simulink model "satellite_model"  (R2024a)
settings: Solver=ode4  StartTime=0.0  StopTime=1500  FixedStep=0.001  RelTol=1e-7  AbsTol=1e-7
values from neighbouring files (symbols this model uses):
  a1 = 5e-6    (= 5e-06)    [quadcopter_param.m]    (also in satellite_param.m = ab1 / I(1,1); unicycle_param.m = 4e-05)
  a2 = 7.5e-6    (= 7.5e-06)    [quadcopter_param.m]    (also in satellite_param.m = ab2 / I(2,2); unicycle_param.m = 0.0052)
  a3 = 8.5e-6    (= 8.5e-06)    [quadcopter_param.m]    (also in satellite_param.m = ab3 / I(3,3))
  a4 = ab1 / -IRW(1,1)    [satellite_param.m]
  a5 = ab2 / -IRW(2,2)    [satellite_param.m]
  a6 = ab3 / -IRW(3,3)    [satellite_param.m]
  c1 = 0.154    [quadcopter_param.m]    (also in satellite_param.m = cb1 / I(1,1); unicycle_param.m = 0.4)
  c2 = 0.237    [quadcopter_param.m]    (also in satellite_param.m = cb2 / I(2,2); unicycle_param.m = 2.4)
  c3 = 0.185    [quadcopter_param.m]    (also in satellite_param.m = cb3 / I(3,3))
  c4 = cb1 / -IRW(1,1)    [satellite_param.m]
  c5 = cb2 / -IRW(2,2)    [satellite_param.m]
  c6 = cb3 / -IRW(3,3)    [satellite_param.m]
  delay = 0.01    [quadcopter_param.m]    (also in satellite_param.m = 0.003; unicycle_param.m)
  k = 3.95    [quadcopter_param.m]    (also in satellite_param.m = 2.4; unicycle_param.m = 12.5)
  omega = 25    [quadcopter_param.m]    (also in satellite_param.m = 36; unicycle_param.m = 50)
  variance = 1e-6    (= 1e-06)    [quadcopter_param.m]    (also in satellite_param.m = 1e-09; unicycle_param.m)
settings Model: Creator=rohan  LastModifiedBy=rohan

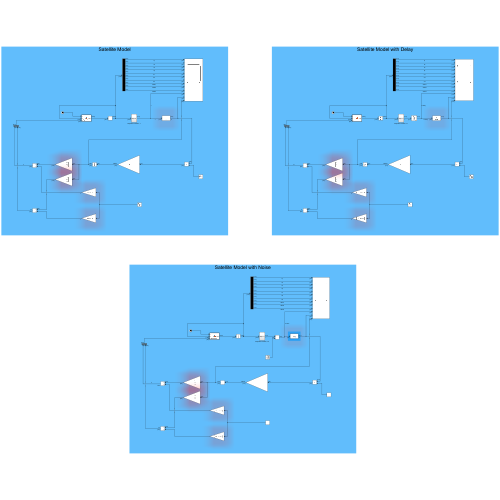
[thumbnail: Simulink's stored preview of the top-level diagram]
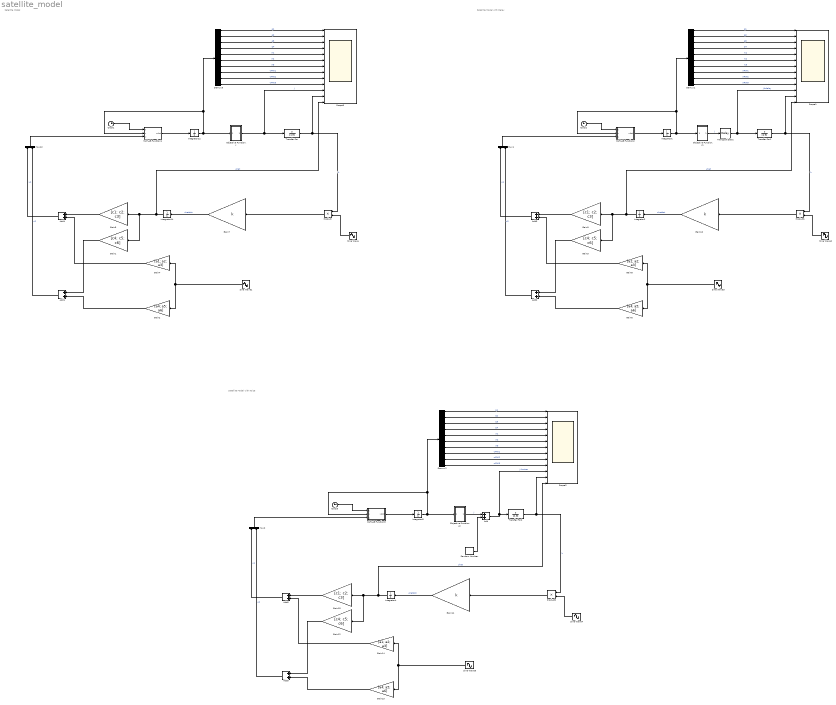
== system satellite_model ==
  note: Satellite Model
  note: Satellite Model with Delay
  note: Satellite Model with Noise
  Add{,1..6} (7 alike) : Sum
  Clock1 : Clock
  Clock2 : Clock
  Clock3 : Clock
  Demux1 : Demux  Outputs=10
  Demux2 : Demux  Outputs=10
  Demux5 : Demux  Outputs=10
  Gain1 : Gain  Gain=[c4; c5; c6]
  Gain10 : Gain  Gain=k
  Gain11 : Gain  Gain=k
  Gain12 : Gain  Gain=[c4; c5; c6]
  Gain13 : Gain  Gain=[a4; a5; a6]
  Gain14 : Gain  Gain=[a1; a2; a3]
  Gain15 : Gain  Gain=[c1; c2; c3]
  Gain2 : Gain  Gain=[a4; a5; a6]
  Gain3 : Gain  Gain=[c4; c5; c6]
  Gain4 : Gain  Gain=[a1; a2; a3]
  Gain5 : Gain  Gain=[c1; c2; c3]
  Gain6 : Gain  Gain=[a4; a5; a6]
  Gain7 : Gain  Gain=k
  Gain8 : Gain  Gain=[a1; a2; a3]
  Gain9 : Gain  Gain=[c1; c2; c3]
  Integrator1 : Integrator  InitialCondition=[0.57; 0.57; 0.57; 0.159; 0.01; 0.01; 0.01; 0; 0; 0]
  Integrator12 : Integrator  InitialCondition=[0.57; 0.57; 0.57; 0.159; 0.01; 0.01; 0.01; 0; 0; 0]
  Integrator14 : Integrator
  Integrator2 : Integrator
  Integrator3 : Integrator  InitialCondition=[0.57; 0.57; 0.57; 0.159; 0.01; 0.01; 0.01; 0; 0; 0]
  Integrator4 : Integrator
  MATLAB Function1 : MATLAB Function  TreatAsAtomicUnit=on
  MATLAB Function2 : MATLAB Function  TreatAsAtomicUnit=on
  MATLAB Function3 : MATLAB Function  TreatAsAtomicUnit=on
  Mux1 : Mux  Inputs=2
  Mux12 : Mux  Inputs=2
  Mux2 : Mux  Inputs=2
  "Objective Function, J" : Subsystem
  "Objective Function, J1" : Subsystem
  "Objective Function, J2" : Subsystem
  Product : Product
  Product1 : Product
  Product2 : Product
  Random Number : RandomNumber  Variance=variance  Seed=1  SampleTime=0.001
  Scope1 : Scope  NumInputPorts=13
  Scope2 : Scope  NumInputPorts=13
  Scope3 : Scope  NumInputPorts=13
  Sine Wave{,1..5} (6 alike) : Sin  Amplitude=omega  Frequency=omega  Phase=pi/2  SampleTime=0
  Transfer Fcn : TransferFcn  Numerator=[1 0]  Denominator=[1 e]
  Transfer Fcn1 : TransferFcn  Numerator=[1 0]  Denominator=[1 e]
  Transfer Fcn2 : TransferFcn  Numerator=[1 0]  Denominator=[1 e]
  Transport Delay : TransportDelay  DelayTime=delay  InitialOutput=3 * (0.57 - 0)^2
  wires:
  MATLAB Function1/1(xdot) -> Integrator12/1
  Integrator12/1 -> MATLAB Function1/2(x), Demux5/1, "Objective Function, J"/1(In2)
  Clock1/1 -> MATLAB Function1/1(t)
  "Objective Function, J"/1(objFun1) -> Transfer Fcn/1, Scope3/11  "J"
  Add4/1 -> Mux12/1  "u1"
  Gain4/1 -> Add4/2
  Integrator14/1 -> Scope3/13, Gain1/1, Gain5/1  "uhat"
  Gain5/1 -> Add4/1
  Sine Wave1/1 -> Gain4/1, Gain2/1
  Sine Wave/1 -> Product/2
  Gain7/1 -> Integrator14/1  "uhatdot"
  Gain1/1 -> Add1/1
  Gain2/1 -> Add1/2
  Add1/1 -> Mux12/2  "u2"
  Mux12/1 -> MATLAB Function1/3(u)
  Demux5/1 -> Scope3/1  "q1"
  Demux5/2 -> Scope3/2  "q2"
  Demux5/3 -> Scope3/3  "q3"
  Demux5/4 -> Scope3/4  "q4"
  Demux5/5 -> Scope3/5  "w1"
  Demux5/6 -> Scope3/6  "w2"
  Demux5/7 -> Scope3/7  "w3"
  Demux5/8 -> Scope3/8  "wRW1"
  Demux5/9 -> Scope3/9  "wRW2"
  Demux5/10 -> Scope3/10  "wRW3"
  Product/1 -> Gain7/1
  Transfer Fcn/1 -> Product/1, Scope3/12  "h"
  Sine Wave2/1 -> Product1/2
  Mux1/1 -> MATLAB Function2/3(u)
  Add2/1 -> Mux1/2  "u2"
  Gain9/1 -> Add3/1
  Gain6/1 -> Add2/2
  Demux1/4 -> Scope1/4  "q4"
  Demux1/9 -> Scope1/9  "wRW2"
  Integrator2/1 -> Scope1/13, Gain3/1, Gain9/1  "uhat"
  Demux1/1 -> Scope1/1  "q1"
  Transfer Fcn1/1 -> Product1/1, Scope1/12  "h"
  Product1/1 -> Gain10/1
  Demux1/7 -> Scope1/7  "w3"
  Demux1/8 -> Scope1/8  "wRW1"
  Demux1/3 -> Scope1/3  "q3"
  Gain3/1 -> Add2/1
  Gain8/1 -> Add3/2
  Demux1/5 -> Scope1/5  "w1"
  Add3/1 -> Mux1/1  "u1"
  "Objective Function, J1"/1(objFun1) -> Transport Delay/1  "J"
  Gain10/1 -> Integrator2/1  "uhatdot"
  Demux1/2 -> Scope1/2  "q2"
  Demux1/10 -> Scope1/10  "wRW3"
  Clock2/1 -> MATLAB Function2/1(t)
  Demux1/6 -> Scope1/6  "w2"
  Integrator1/1 -> MATLAB Function2/2(x), Demux1/1, "Objective Function, J1"/1(In2)
  MATLAB Function2/1(xdot) -> Integrator1/1
  Sine Wave3/1 -> Gain8/1, Gain6/1
  Sine Wave5/1 -> Gain13/1, Gain14/1
  MATLAB Function3/1(xdot) -> Integrator3/1
  Integrator3/1 -> "Objective Function, J2"/1(In2), Demux2/1, MATLAB Function3/2(x)
  Demux2/6 -> Scope2/6  "w2"
  Clock3/1 -> MATLAB Function3/1(t)
  Demux2/10 -> Scope2/10  "wRW3"
  Demux2/2 -> Scope2/2  "q2"
  Gain11/1 -> Integrator4/1  "uhatdot"
  Add6/1 -> Mux2/1  "u1"
  Demux2/5 -> Scope2/5  "w1"
  Gain14/1 -> Add6/2
  Gain12/1 -> Add5/1
  Demux2/3 -> Scope2/3  "q3"
  Demux2/8 -> Scope2/8  "wRW1"
  Demux2/7 -> Scope2/7  "w3"
  Product2/1 -> Gain11/1
  Transfer Fcn2/1 -> Scope2/12, Product2/1  "h"
  Demux2/1 -> Scope2/1  "q1"
  Integrator4/1 -> Scope2/13, Gain15/1, Gain12/1  "uhat"
  Demux2/9 -> Scope2/9  "wRW2"
  Demux2/4 -> Scope2/4  "q4"
  Gain13/1 -> Add5/2
  Gain15/1 -> Add6/1
  Add5/1 -> Mux2/2  "u2"
  Mux2/1 -> MATLAB Function3/3(u)
  Sine Wave4/1 -> Product2/2
  Transport Delay/1 -> Transfer Fcn1/1, Scope1/11  "J+delay"
  "Objective Function, J2"/1(objFun1) -> Add/1  "J"
  Add/1 -> Transfer Fcn2/1, Scope2/11  "J+noise"
  Random Number/1 -> Add/2

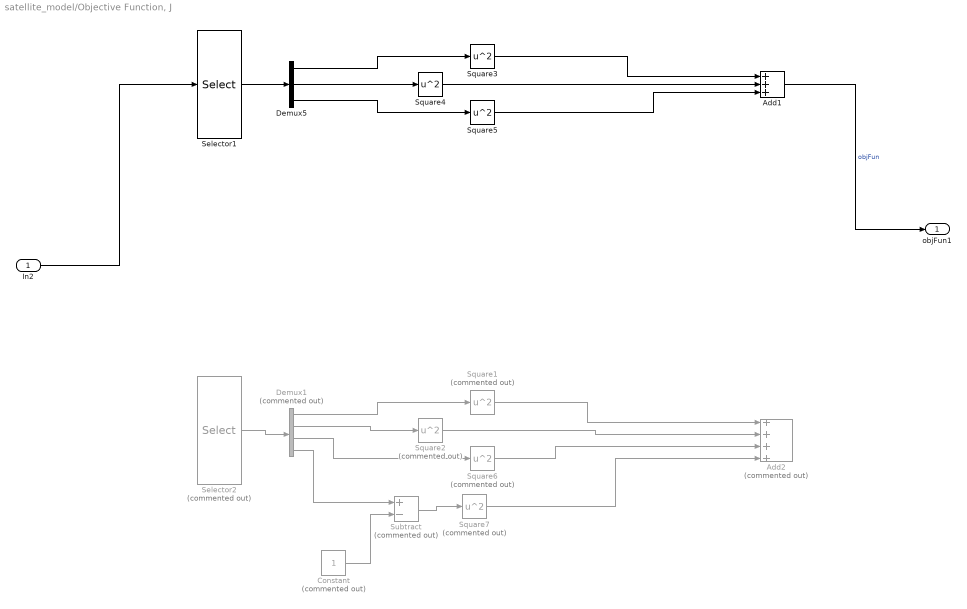
== system satellite_model/Objective Function, J ==
  In2 : Inport
  Add1 : Sum  Inputs=+++
  Add2 : Sum  Commented=on  Inputs=++++
  Constant : Constant  Commented=on
  Demux1 : Demux  Commented=on
  Demux5 : Demux  Outputs=3
  Selector1 : Selector  InputPortWidth=10  IndexOptions=Index vector (dialog)  Indices=[1 2 3]  OutputSizes=1
  Selector2 : Selector  Commented=on  InputPortWidth=10  IndexOptions=Index vector (dialog)  Indices=[1 2 3 4]  OutputSizes=1
  Square{1..2,6..7} (4 alike) : Math  Commented=on  Operator=square
  Square3 : Math  Operator=square
  Square4 : Math  Operator=square
  Square5 : Math  Operator=square
  Subtract : Sum  Commented=on  Inputs=+-
  objFun1 : Outport
  wires:
  Square4/1 -> Add1/2
  Demux5/2 -> Square4/1
  Square5/1 -> Add1/3
  Demux5/1 -> Square3/1
  Selector1/1 -> Demux5/1
  Square3/1 -> Add1/1
  Demux5/3 -> Square5/1
  Demux1/3 -> Square6/1
  Square1/1 -> Add2/1
  Selector2/1 -> Demux1/1
  Demux1/1 -> Square1/1
  Square6/1 -> Add2/3
  Demux1/2 -> Square2/1
  Square2/1 -> Add2/2
  Demux1/4 -> Subtract/1
  Constant/1 -> Subtract/2
  Subtract/1 -> Square7/1
  Square7/1 -> Add2/4
  In2/1 -> Selector1/1
  Add1/1 -> objFun1/1  "objFun"

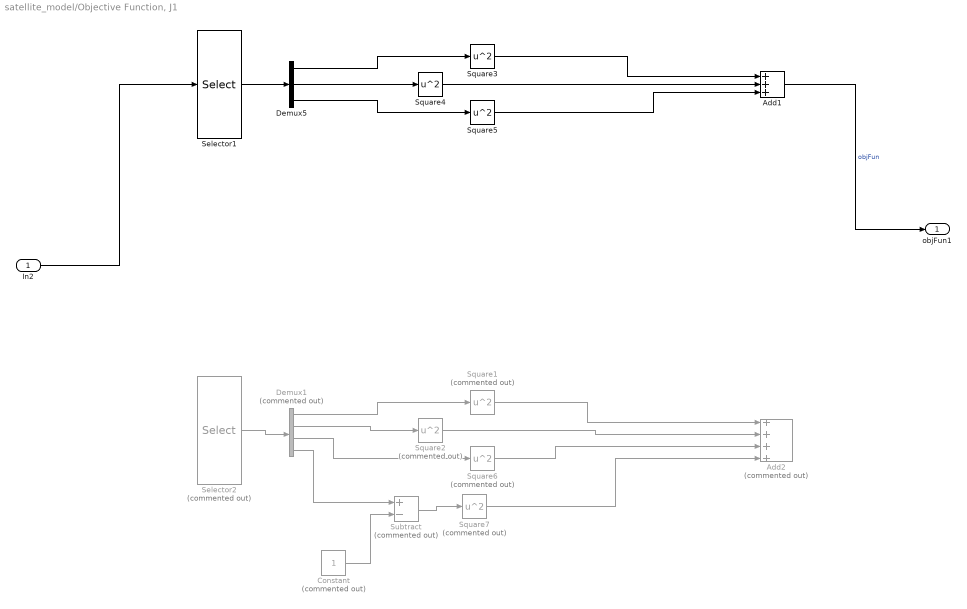
== system satellite_model/Objective Function, J1 ==
  In2 : Inport
  Add1 : Sum  Inputs=+++
  Add2 : Sum  Commented=on  Inputs=++++
  Constant : Constant  Commented=on
  Demux1 : Demux  Commented=on
  Demux5 : Demux  Outputs=3
  Selector1 : Selector  InputPortWidth=10  IndexOptions=Index vector (dialog)  Indices=[1 2 3]  OutputSizes=1
  Selector2 : Selector  Commented=on  InputPortWidth=10  IndexOptions=Index vector (dialog)  Indices=[1 2 3 4]  OutputSizes=1
  Square{1..2,6..7} (4 alike) : Math  Commented=on  Operator=square
  Square3 : Math  Operator=square
  Square4 : Math  Operator=square
  Square5 : Math  Operator=square
  Subtract : Sum  Commented=on  Inputs=+-
  objFun1 : Outport
  wires:
  Square4/1 -> Add1/2
  Demux5/2 -> Square4/1
  Square5/1 -> Add1/3
  Demux5/1 -> Square3/1
  Selector1/1 -> Demux5/1
  Square3/1 -> Add1/1
  Demux5/3 -> Square5/1
  Demux1/3 -> Square6/1
  Square1/1 -> Add2/1
  Selector2/1 -> Demux1/1
  Demux1/1 -> Square1/1
  Square6/1 -> Add2/3
  Demux1/2 -> Square2/1
  Square2/1 -> Add2/2
  Demux1/4 -> Subtract/1
  Constant/1 -> Subtract/2
  Subtract/1 -> Square7/1
  Square7/1 -> Add2/4
  In2/1 -> Selector1/1
  Add1/1 -> objFun1/1  "objFun"

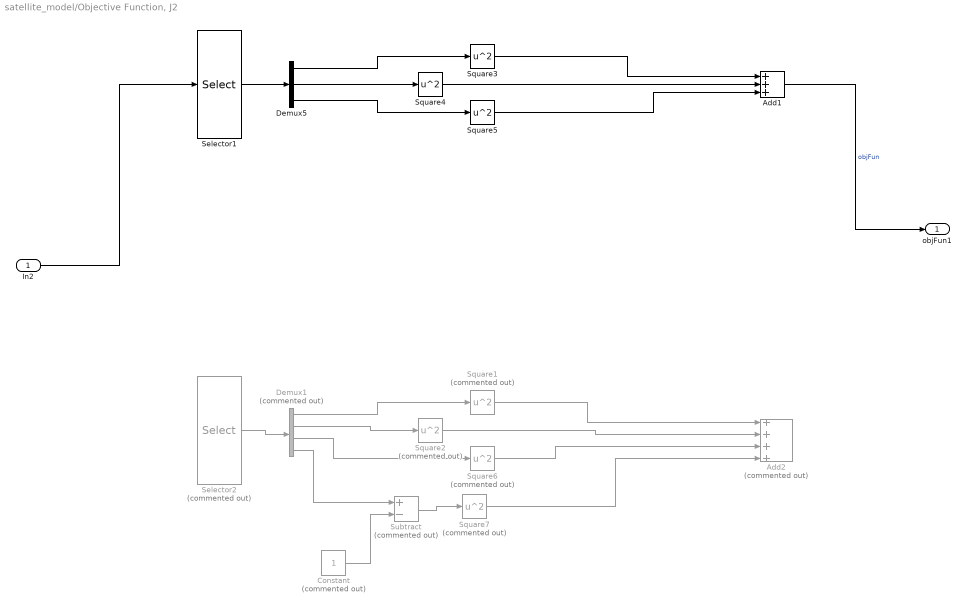
== system satellite_model/Objective Function, J2 ==
  In2 : Inport
  Add1 : Sum  Inputs=+++
  Add2 : Sum  Commented=on  Inputs=++++
  Constant : Constant  Commented=on
  Demux1 : Demux  Commented=on
  Demux5 : Demux  Outputs=3
  Selector1 : Selector  InputPortWidth=10  IndexOptions=Index vector (dialog)  Indices=[1 2 3]  OutputSizes=1
  Selector2 : Selector  Commented=on  InputPortWidth=10  IndexOptions=Index vector (dialog)  Indices=[1 2 3 4]  OutputSizes=1
  Square{1..2,6..7} (4 alike) : Math  Commented=on  Operator=square
  Square3 : Math  Operator=square
  Square4 : Math  Operator=square
  Square5 : Math  Operator=square
  Subtract : Sum  Commented=on  Inputs=+-
  objFun1 : Outport
  wires:
  Add1/1 -> objFun1/1  "objFun"
  In2/1 -> Selector1/1
  Square7/1 -> Add2/4
  Subtract/1 -> Square7/1
  Constant/1 -> Subtract/2
  Demux1/4 -> Subtract/1
  Square2/1 -> Add2/2
  Demux1/2 -> Square2/1
  Square6/1 -> Add2/3
  Demux1/1 -> Square1/1
  Selector2/1 -> Demux1/1
  Square1/1 -> Add2/1
  Demux1/3 -> Square6/1
  Demux5/3 -> Square5/1
  Square3/1 -> Add1/1
  Selector1/1 -> Demux5/1
  Demux5/1 -> Square3/1
  Square5/1 -> Add1/3
  Demux5/2 -> Square4/1
  Square4/1 -> Add1/2

== matlab function satellite_model/MATLAB Function2 ==
  data: t input; x input; u input; xdot output
function xdot = dynamics(t,x,u)

q1 = x(1); q2 = x(2); q3 = x(3); q4 = x(4);
w1 = x(5); w2 = x(6); w3 = x(7);
wRW1 = x(8); wRW2 = x(9); wRW3 = x(10);

u1 = u(1:3);
u2 = u(4:6);

% Parameters
I = diag([1, 2, 3]);
IRW = 0.005 * eye(3);

r1 = I(1,1)/5; r2 = I(2,2)/5; r3 = I(3,3)/5;


A = [q4 -q3 q2;
     q3 q4 -q1;
     -q2 q1 q4;
     -q1 -q2 -q3];

wArray = [w1; w2; w3];
wSkewSym = [0 -w3 w2;
            w3 0 -w1;
            -w2 w1 0];
R = diag([r1, r2, r3]);

wRWArray = [wRW1; wRW2; wRW3];

qdot = 1/2 * A * wArray;
wdot = I\(-wSkewSym*(I*wArray) - wSkewSym*(IRW*wRWArray) - R*wArray) + u1;
wRWdot = u2;


xdot = [qdot; wdot; wRWdot];

== matlab function satellite_model/MATLAB Function3 ==
  data: t input; x input; u input; xdot output
function xdot = dynamics(t,x,u)

q1 = x(1); q2 = x(2); q3 = x(3); q4 = x(4);
w1 = x(5); w2 = x(6); w3 = x(7);
wRW1 = x(8); wRW2 = x(9); wRW3 = x(10);

u1 = u(1:3);
u2 = u(4:6);

% Parameters
I = diag([1, 2, 3]);
IRW = 0.005 * eye(3);

r1 = I(1,1)/5; r2 = I(2,2)/5; r3 = I(3,3)/5;


A = [q4 -q3 q2;
     q3 q4 -q1;
     -q2 q1 q4;
     -q1 -q2 -q3];

wArray = [w1; w2; w3];
wSkewSym = [0 -w3 w2;
            w3 0 -w1;
            -w2 w1 0];
R = diag([r1, r2, r3]);

wRWArray = [wRW1; wRW2; wRW3];

qdot = 1/2 * A * wArray;
wdot = I\(-wSkewSym*(I*wArray) - wSkewSym*(IRW*wRWArray) - R*wArray) + u1;
wRWdot = u2;


xdot = [qdot; wdot; wRWdot];

== matlab function satellite_model/MATLAB Function1 ==
  data: t input; x input; u input; xdot output
function xdot = dynamics(t,x,u)

q1 = x(1); q2 = x(2); q3 = x(3); q4 = x(4);
w1 = x(5); w2 = x(6); w3 = x(7);
wRW1 = x(8); wRW2 = x(9); wRW3 = x(10);

u1 = u(1:3);
u2 = u(4:6);

% Parameters
I = diag([1, 2, 3]);
IRW = 0.005 * eye(3);

r1 = I(1,1)/5; r2 = I(2,2)/5; r3 = I(3,3)/5;


A = [q4 -q3 q2;
     q3 q4 -q1;
     -q2 q1 q4;
     -q1 -q2 -q3];

wArray = [w1; w2; w3];
wSkewSym = [0 -w3 w2;
            w3 0 -w1;
            -w2 w1 0];
R = diag([r1, r2, r3]);

wRWArray = [wRW1; wRW2; wRW3];

qdot = 1/2 * A * wArray;
wdot = I\(-wSkewSym*(I*wArray) - wSkewSym*(IRW*wRWArray) - R*wArray) + u1;
wRWdot = u2;


xdot = [qdot; wdot; wRWdot];
